simulink model "CenterMass"  (R2018b)
settings: Solver=VariableStepAuto  StartTime=0.0  StopTime=10.0  RelTol=1e-3
settings Model: Creator=Yahya  LastModifiedBy=Yahya

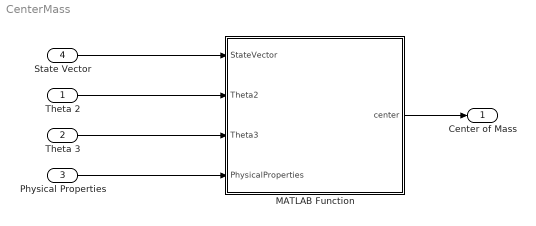
== system CenterMass ==
  Theta 2 : Inport
  Theta 3 : Inport  Port=2
  Physical Properties : Inport  Port=3  PortDimensions=6
  State Vector : Inport  Port=4  PortDimensions=2
  MATLAB Function : MATLAB Function  TreatAsAtomicUnit=on
  Center of Mass : Outport  PortDimensions=1
  wires:
  Physical Properties/1 -> MATLAB Function/4(PhysicalProperties)
  Theta 3/1 -> MATLAB Function/3(Theta3)
  Theta 2/1 -> MATLAB Function/2(Theta2)
  State Vector/1 -> MATLAB Function/1(StateVector)
  MATLAB Function/1(center) -> Center of Mass/1

== matlab function CenterMass/MATLAB Function ==
  data: StateVector input; center output; Theta2 input; Theta3 input; PhysicalProperties input
function center = CenterMass(StateVector, Theta2, Theta3, PhysicalProperties)

center = CMcalculator(StateVector, Theta2, Theta3, PhysicalProperties);

end
